simulink subsystem "LP_First_Order"  (R2024b)
settings: Solver=VariableStepAuto  StartTime=0.0  StopTime=10.0  RelTol=1e-3
settings Model: Creator=mykola  LastModifiedBy=mykola

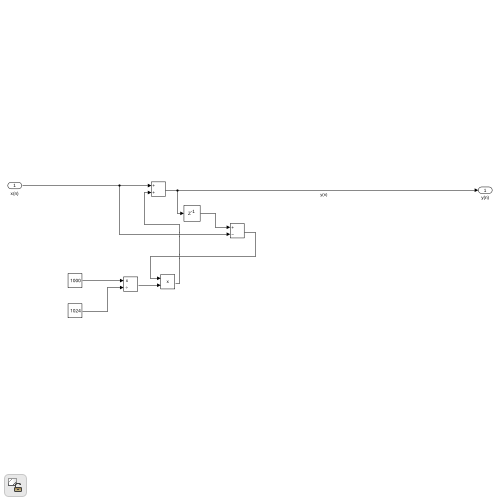
[thumbnail: Simulink's stored preview of the top-level diagram]
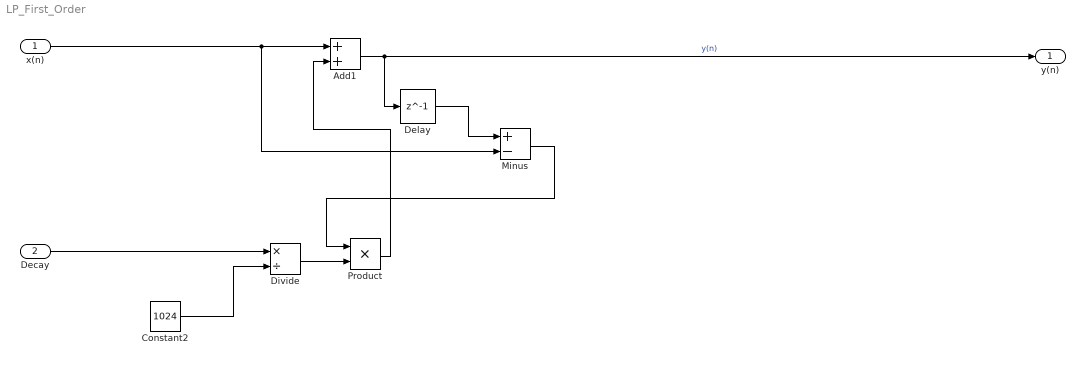
== system LP_First_Order ==
  x(n) : Inport
  Decay : Inport  Port=2
  Add1 : Sum
  Constant2 : Constant  Value=1024
  Delay : Delay  DelayLength=1
  Divide : Product  Inputs=*/
  Minus : Sum  Inputs=+-
  Product : Product
  y(n) : Outport
  wires:
  Divide/1 -> Product/2
  Constant2/1 -> Divide/2
  Product/1 -> Add1/2
  Decay/1 -> Divide/1
  Minus/1 -> Product/1
  Delay/1 -> Minus/1
  x(n)/1 -> Add1/1, Minus/2
  Add1/1 -> Delay/1, y(n)/1  "y(n)"
